simulink model "Simulink_Mega"  (R2021b)
settings: Solver=VariableStepAuto  StartTime=0.0  StopTime=10.0  RelTol=1e-3
InitFcn:
  | encoderCounter1 = 0;
  | encoderCounter2 = 0;
  | encoderMapped1 = 0;
  | encoderMapped2 = 0;
values from neighbouring files (symbols this model uses):
  PULSE_PER_REV = 1200    [Matlab_Mega_Init.m]
libraries: arduinolib x11, simulink x2
settings Model: Creator=james  LastModifiedBy=james

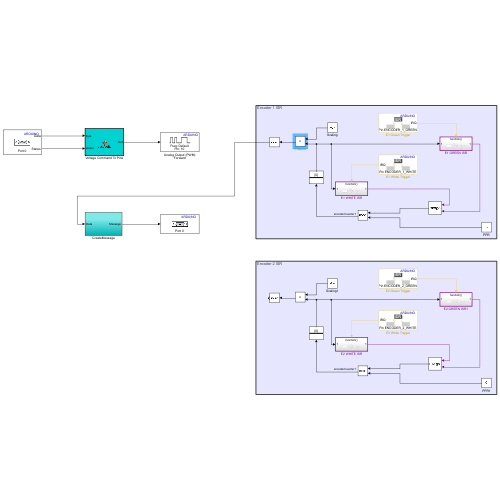
[thumbnail: Simulink's stored preview of the top-level diagram]
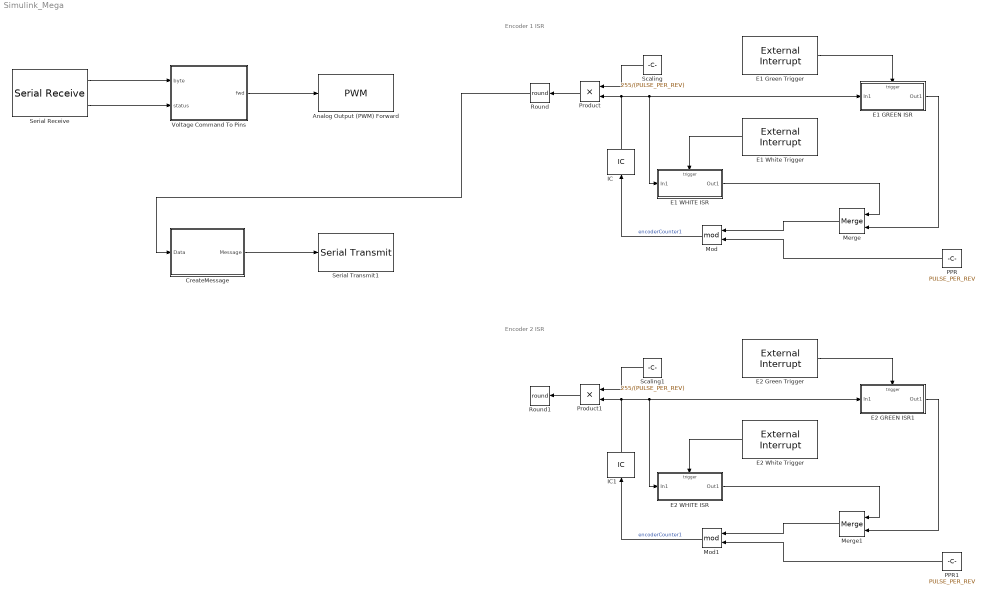
== system Simulink_Mega ==
  note: Encoder 1 ISR
  note: Encoder 2 ISR
  Analog Output (PWM) Forward : arduinolib/PWM  pinNumber=10  frequencyType=Default  desiredFrequency=490.2  achievableFrequency=490.2
  CreateMessage : Subsystem
  E1 GREEN ISR : Subsystem  TreatAsAtomicUnit=on
  E1 Green Trigger : arduinolib/External Interrupt  Pin=ENCODER_1_GREEN  PullUp=on  Mode=RISING  InterruptSimulationInput=off
      settings: SourceProductBaseCode=ARDUINO
  E1 WHITE ISR : Subsystem  TreatAsAtomicUnit=on
  E1 White Trigger : arduinolib/External Interrupt  Pin=ENCODER_1_WHITE  PullUp=on  Mode=RISING  InterruptSimulationInput=off
      settings: SourceProductBaseCode=ARDUINO
  E2 GREEN ISR1 : Subsystem  TreatAsAtomicUnit=on
  E2 Green Trigger : arduinolib/External Interrupt  Pin=ENCODER_2_GREEN  PullUp=on  Mode=RISING  InterruptSimulationInput=off
      settings: SourceProductBaseCode=ARDUINO
  E2 WHITE ISR : Subsystem  TreatAsAtomicUnit=on
  E2 White Trigger : arduinolib/External Interrupt  Pin=ENCODER_2_WHITE  PullUp=on  Mode=RISING  InterruptSimulationInput=off
      settings: SourceProductBaseCode=ARDUINO
  IC : InitialCondition  Value=0
  IC1 : InitialCondition  Value=0
  Merge : Merge  InitialOutput=[0]
  Merge1 : Merge  InitialOutput=[0]
  Mod : Math  Operator=mod  SaturateOnIntegerOverflow=on
  Mod1 : Math  Operator=mod  SaturateOnIntegerOverflow=on
  PPR : Constant  Value=PULSE_PER_REV
  PPR1 : Constant  Value=PULSE_PER_REV
  Product : Product
  Product1 : Product
  Round : Rounding  Operator=round
  Round1 : Rounding  Operator=round
  Scaling : Constant  Value=255/(PULSE_PER_REV)
  Scaling1 : Constant  Value=255/(PULSE_PER_REV)
  Serial Receive : arduinolib/Serial Receive  isARMArch=off  portNumber=0  DataType=uint8  Datalength=1  SampleTime=0.01  showOutStatus=on  blockPlatform=arduino
      settings: SourceProductBaseCode=ARDUINO
  Serial Transmit1 : arduinolib/Serial Transmit  portNumber=0  sendmode=write  sendformat=Decimal  floatprecision=2  blockPlatform=arduino
  Voltage Command To Pins : MATLAB Function  TreatAsAtomicUnit=on
  wires:
  E1 White Trigger/1 -> E1 WHITE ISR/Trigger
  E1 WHITE ISR/1(Out1) -> Merge/1
  IC/1 -> Product/2, E1 WHITE ISR/1(In1), E1 GREEN ISR/1(In1)
  Mod/1 -> IC/1  "encoderCounter1"
  E1 Green Trigger/1 -> E1 GREEN ISR/Trigger
  PPR/1 -> Mod/2
  E1 GREEN ISR/1(Out1) -> Merge/2
  Merge/1 -> Mod/1
  Product/1 -> Round/1
  Scaling/1 -> Product/1
  Scaling1/1 -> Product1/1
  Product1/1 -> Round1/1
  Merge1/1 -> Mod1/1
  E2 GREEN ISR1/1(Out1) -> Merge1/2
  PPR1/1 -> Mod1/2
  E2 Green Trigger/1 -> E2 GREEN ISR1/Trigger
  Mod1/1 -> IC1/1  "encoderCounter1"
  IC1/1 -> E2 GREEN ISR1/1(In1), E2 WHITE ISR/1(In1), Product1/2
  E2 WHITE ISR/1(Out1) -> Merge1/1
  E2 White Trigger/1 -> E2 WHITE ISR/Trigger
  Serial Receive/1 -> Voltage Command To Pins/1(byte)
  Serial Receive/2 -> Voltage Command To Pins/2(status)
  Round/1 -> CreateMessage/1(Data)
  Voltage Command To Pins/1(fwd) -> Analog Output (PWM) Forward/1
  CreateMessage/1(Message) -> Serial Transmit1/1

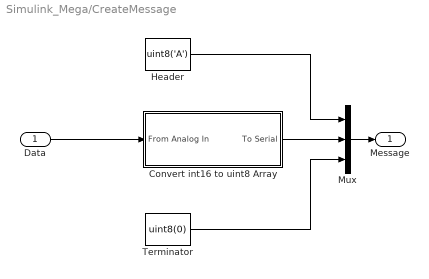
== system Simulink_Mega/CreateMessage ==
  Data : Inport
  Convert int16 to uint8 Array : Subsystem
  Header : Constant  Value=uint8('A')
  Mux : Mux  Inputs=3
  Terminator : Constant  Value=uint8(0)
  Message : Outport
  wires:
  Header/1 -> Mux/1
  Terminator/1 -> Mux/3
  Data/1 -> Convert int16 to uint8 Array/1(From Analog In)
  Mux/1 -> Message/1
  Convert int16 to uint8 Array/1(To Serial) -> Mux/2

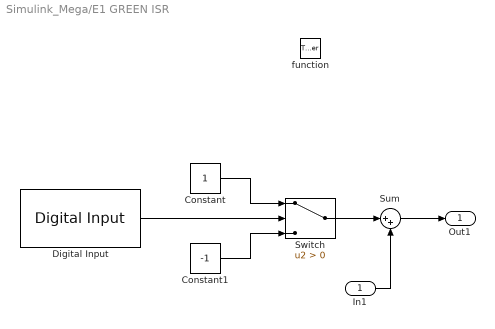
== system Simulink_Mega/E1 GREEN ISR ==
  In1 : Inport
  function : TriggerPort  TriggerType=function-call  VariantControl=Variant
  Constant : Constant
  Constant1 : Constant  Value=-1
  Digital Input : arduinolib/Digital Input  pinNumber=ENCODER_1_WHITE  mode=Input Pullup  Direction=input  SampleTime=0.1  blockPlatform=arduino
  Sum : Sum  Inputs=|++
  Switch : Switch  Criteria=u2 > Threshold
  Out1 : Outport  VectorParamsAs1DForOutWhenUnconnected=off
  wires:
  Switch/1 -> Sum/1
  Sum/1 -> Out1/1
  In1/1 -> Sum/2
  Constant1/1 -> Switch/3
  Constant/1 -> Switch/1
  Digital Input/1 -> Switch/2

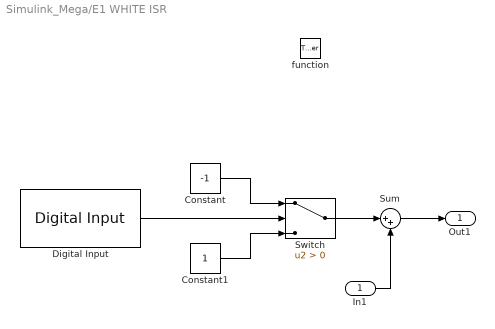
== system Simulink_Mega/E1 WHITE ISR ==
  In1 : Inport
  function : TriggerPort  TriggerType=function-call  VariantControl=Variant
  Constant : Constant  Value=-1
  Constant1 : Constant
  Digital Input : arduinolib/Digital Input  pinNumber=ENCODER_1_GREEN  mode=Input Pullup  Direction=input  SampleTime=0.1  blockPlatform=arduino
  Sum : Sum  Inputs=|++
  Switch : Switch  Criteria=u2 > Threshold
  Out1 : Outport  VectorParamsAs1DForOutWhenUnconnected=off
  wires:
  Digital Input/1 -> Switch/2
  Constant/1 -> Switch/1
  Constant1/1 -> Switch/3
  In1/1 -> Sum/2
  Sum/1 -> Out1/1
  Switch/1 -> Sum/1

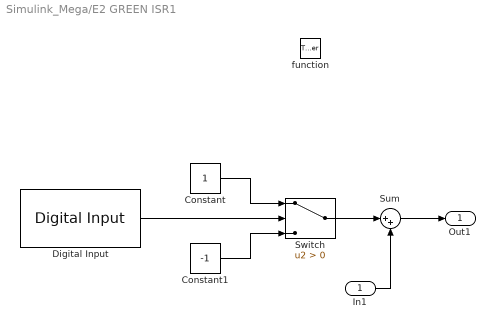
== system Simulink_Mega/E2 GREEN ISR1 ==
  In1 : Inport
  function : TriggerPort  TriggerType=function-call  VariantControl=Variant
  Constant : Constant
  Constant1 : Constant  Value=-1
  Digital Input : arduinolib/Digital Input  pinNumber=ENCODER_2_WHITE  mode=Input Pullup  Direction=input  SampleTime=0.1  blockPlatform=arduino
  Sum : Sum  Inputs=|++
  Switch : Switch  Criteria=u2 > Threshold
  Out1 : Outport  VectorParamsAs1DForOutWhenUnconnected=off
  wires:
  Digital Input/1 -> Switch/2
  Constant/1 -> Switch/1
  Constant1/1 -> Switch/3
  In1/1 -> Sum/2
  Sum/1 -> Out1/1
  Switch/1 -> Sum/1

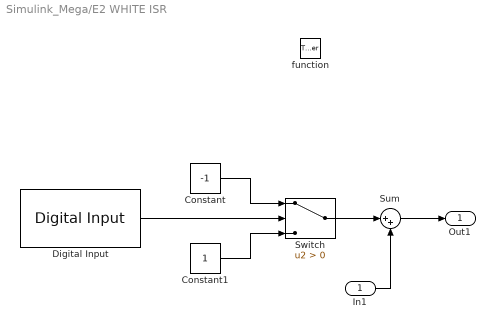
== system Simulink_Mega/E2 WHITE ISR ==
  In1 : Inport
  function : TriggerPort  TriggerType=function-call  VariantControl=Variant
  Constant : Constant  Value=-1
  Constant1 : Constant
  Digital Input : arduinolib/Digital Input  pinNumber=ENCODER_2_GREEN  mode=Input Pullup  Direction=input  SampleTime=0.1  blockPlatform=arduino
  Sum : Sum  Inputs=|++
  Switch : Switch  Criteria=u2 > Threshold
  Out1 : Outport  VectorParamsAs1DForOutWhenUnconnected=off
  wires:
  Switch/1 -> Sum/1
  Sum/1 -> Out1/1
  In1/1 -> Sum/2
  Constant1/1 -> Switch/3
  Constant/1 -> Switch/1
  Digital Input/1 -> Switch/2

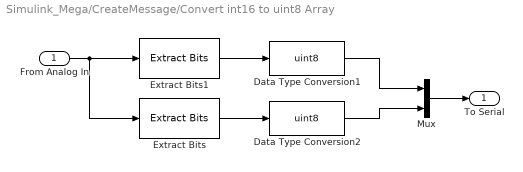
== system Simulink_Mega/CreateMessage/Convert int16 to uint8 Array ==
  From Analog In : Inport
  Data Type Conversion1 : DataTypeConversion  OutDataTypeStr=uint8  ConvertRealWorld=Stored Integer (SI)
  Data Type Conversion2 : DataTypeConversion  OutDataTypeStr=uint8  ConvertRealWorld=Stored Integer (SI)
  Extract Bits : simulink/Logic and Bit Operations/Extract Bits  bitsToExtract=Upper half  numBits=8  bitIdxRange=[0 7]  outScalingMode=Treat bit field as an integer
  Extract Bits1 : simulink/Logic and Bit Operations/Extract Bits  bitsToExtract=Lower half  numBits=8  bitIdxRange=[0 7]  outScalingMode=Treat bit field as an integer
  Mux : Mux  Inputs=2
  To Serial : Outport
  wires:
  Extract Bits/1 -> Data Type Conversion2/1
  Extract Bits1/1 -> Data Type Conversion1/1
  From Analog In/1 -> Extract Bits1/1, Extract Bits/1
  Mux/1 -> To Serial/1
  Data Type Conversion1/1 -> Mux/1
  Data Type Conversion2/1 -> Mux/2

== matlab function Simulink_Mega/Voltage Command To Pins ==
  data: byte input; fwd output; status input
function fwd  = passVolts(byte,status)
%#codegen
persistent last

if isempty(last)
    last = int16(0);
end

if (byte>=0 && status == 1)
    volt = int16(byte);
    last = volt;
else
    volt = last;
end

fwd = uint8(volt);

end
